simulink model "webserver_demo"  (Simulink 7.3)
settings: Solver=FixedStepDiscrete  SolverMode=SingleTasking  StartTime=0.0  StopTime=10.0  RelTol=1e-3
PreLoadFcn:
  | waijung.modelPreload; % Required for working with Waijung Blockset. Do not remove.
undefined symbols (not defined in the file): A1, A2, A7, B10, B11, B12, Blocking, C1, C2, C3, C4, C5, G14, GPIO_Pin_13, H2, H3, H6, H7, HSEOSC, Link, LQFP176, Non, ST, STM32F417IG
libraries: simulink x14, stm32f4_io_lib x4, waijung_webserver x3, amg_sqlite_dataserver x3, stm32f4_adc_lib x1, stm32f4_device_config_lib x1
(part 2 of 3)

== system webserver_demo/Http Webserver Setup ==
  Ethernet Application Setup : waijung_webserver/Ethernet Application Setup  conf=Setup  ipaddress=192.168.1.41  netmask=255.255.255.0  gateway=192.168.1.1  macaddress=02-00-00-00-00-00  dhcp=off  timerscaler=10  portpinstr=0  sampletime=0.001  blockid=HttpWebserverSetupEthernetApplicationSetup  inputporttype=[]  inputportwidth=[]  inputportlabel={}  outputporttype=[]  outputportwidth=[]  outputportlabel={}  compat=0  optionstring="[\"Dummy\",\"192\",\"168\",\"1\",\"41\",\"255\",\"255\",\"255\",\"0\",\"192\",\"168\",\"1\",\"1\",\"02\",\"00\",\"00\",\"00\",\"00\",\"00\",\"off\",\"10\"]"
  Ethernet Link Setup : waijung_webserver/Ethernet Link Setup  conf=Setup  interfacepin=Profile #2  wj_interfacetype=MII  pin_mdio=A2  pin_mdc=C1  pin_pps=Not used  pin_crs=H2  pin_col=H3  pin_dv=A7  pin_rxclk=A1  pin_rxer=B10  pin_rxd0=C4  pin_rxd1=C5  pin_rxd2=H6  pin_rxd3=H7  pin_txclk=C3  pin_txen=B11  pin_txd0=B12  pin_txd1=G14  pin_txd2=C2  pin_txd3=E2  portpinstr=H2,A1,A2,H3,A7,H6,H7,E2,B10,B11,B12,G14,C1,C2,C3,C4,C5  sampletime=inf  blockid=HttpWebserverSetupEthernetLinkSetup  inputporttype=[]  inputportwidth=[]  inputportlabel={}  outputporttype=[]  outputportwidth=[]  outputportlabel={}  compat=0  optionstring="[\"xxx\",\"on\",\"on\",\"on\",\"off\",\"on\",\"off\",\"on\",\"on\",\"off\",\"on\",\"on\",\"on\",\"on\",\"on\",\"on\",\"on\",\"off\",\"on\",\"on\",\"on\",\"on\",\"on\",\"on\",\"on\",\"on\",\"on\",\"on\",\"H\",\"2\",\"A\",\"1\",\"A\",\"2\",\"H\",\"3\",\"A\",\"7\",\"H\",\"6\",\"H\",\"7\",\"N\",\"ot used\",\"E\",\"2\",\"B\",\"10\",\"B\",\"11\",\"B\",\"12\",\"G\",\"14\",\"C\",\"1\",\"C\",\"2\",\"C\",\"3\",\"C\",\"4\",\"C\",\"5\",\"MII\"]"
  Http Server Setup : waijung_webserver/Http Server Setup  conf=Setup  port=80  ssl=Disable  sqlite=Enable  iap=Disable  mempool=8  debugport=Disable  portpinstr=0  sampletime=inf  blockid=HttpWebserverSetupHttpServerSetup  inputporttype=[]  inputportwidth=[]  inputportlabel={}  outputporttype=[]  outputportwidth=[]  outputportlabel={}  compat=0  optionstring="[\"80\",\"0\",\"0\",\"Enable\",\"Disable\",\"8\",\"17.02a\",\"\",\"\",\"\",\"adc\",\"single\",\"ADCDemoVolatileDataStorage2_adc\",\"1\",\"0\",\"0\",\"(void*)0\",\"%1.2f\",\"\",\"\",\"adc_f\",\"string\",\"ADCDemoVolatileDataStorage3_adc_f\",\"64\",\"0\",\"0\",\"(void*)0\",\"%s\",\"\",\"\",\"btn2\",\"string\",\"ButtonDemoVolatileDataStorage2_btn2\",\"4\",\"0\",\"0\",\"(void*)0\",\"%s\",\"\",\"\",\"btn3\",\"string\",\"ButtonDemoVolatileDataStorage3_btn3\",\"4\",\"0\",\"0\",\"(void*)0\",\"%s\",\"\",\"\",\"btn1\",\"string\",\"ButtonDemoVolatileDataStorage5_btn1\",\"4\",\"0\",\"0\",\"(void*)0\",\"%s\",\"\",\"\",\"dip\",\"string\",\"DIPSwitchDemoVolatileDataStorage_dip\",\"64\",\"1\",\"0\",\"(void*)0\",\"%s\",\"\",\"\",\"datetime\",\"string\",\"HighprecisionRTCDemoVolatileDataStorage1_datetime\",\"64\",\"1\",\"0\",\"(void*)0\",\"%s\",\"\",\"\",\"lcd_line2\",\"string\",\"LCDDemoVolatileDataStorage1_lcd_line2\",\"17\",\"1\",\"0\",\"(void*)0\",\"%s\",\"\",\"\",\"lcd_line3\",\"string\",\"LCDDemoVolatileDataStorage2_lcd_line3\",\"17\",\"1\",\"0\",\"(void*)0\",\"%s\",\"\",\"\",\"lcd_line4\",\"string\",\"LCDDemoVolatileDataStorage3_lcd_line4\",\"17\",\"1\",\"0\",\"(void*)0\",\"%s\",\"\",\"\",\"lcd_line1\",\"string\",\"LCDDemoVolatileDataStorage4_lcd_line1\",\"17\",\"1\",\"0\",\"(void*)0\",\"%s\",\"\",\"\",\"led1\",\"uint32\",\"LEDToggleDemoVolatileDataStorage_led1\",\"1\",\"1\",\"0\",\"LEDToggleDemoHttpserverCGIvarsetcallback_varset_ISR\",\"%u\",\"\",\"\",\"pwm\",\"uint32\",\"PWMDemoVolatileDataStorage_pwm\",\"1\",\"1\",\"0\",\"(void*)0\",\"%u\",\"\",\"\"]"

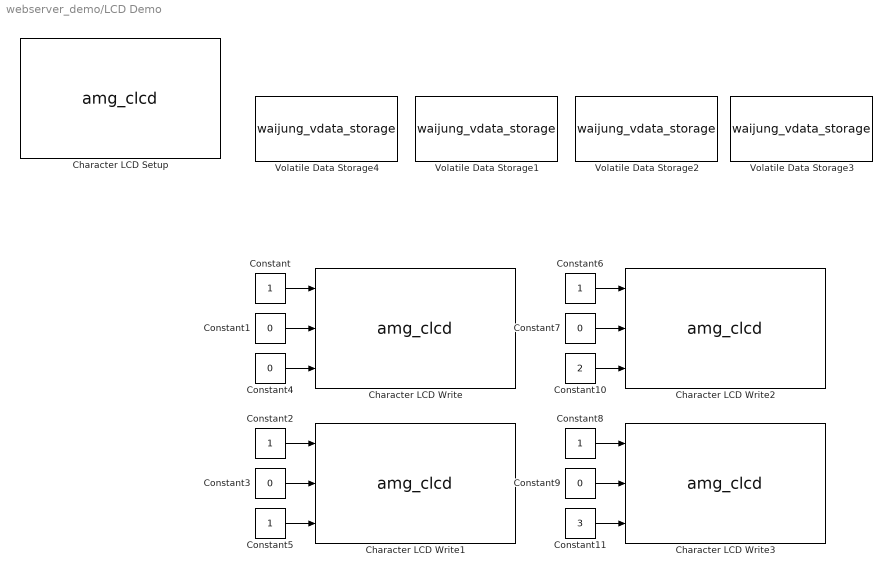
== system webserver_demo/LCD Demo ==
  Character LCD Setup : S-Function  FunctionName=amg_clcd  Parameters=module,configuration,inputtypearray,outputtypearray,confstr,sampletime,sampletimestr,blockid  EnableBusSupport=off  mask(amg_clcd){configuration=Setup, module=1, model=amg CLCD Std, interface=4-bits, linecount=4, columncount=16, gpiotype=Push-pull, controlport=E, control_rs=7, control_rw=8, control_en=9, dataport=E, data0=12, data1=13, data2=14, data3=15, usestringbuffer=off, stringbuffer=<empty>, varname=, inputtypearray=[0], outputtypearray=[0], confstr=["4","4","16","PP","E","7","9","8","","E","","","","","12","13","14","15","0","","0","0","0","0","1","0","0","0","0","stm32f4"], sampletime=-1, sampletimestr=0.001, blockid=LCDDemoCharacterLCDSetup}
      mask prompts: model "LCD model:"; linecount "Number of lines (2 or 4):"; columncount "Number of columns:"; gpiotype "GPIO Output type:"; controlport "GPIO control port:"; control_rs "GPIO control pin, RS:"; control_rw "GPIO control pin, RW:"; control_en "GPIO control pin, EN:"; dataport "GPIO data D[7:4] port"; data0 "GPIO data pin, D4:"; data1 "GPIO data pin, D5:"; data2 "GPIO data pin, D6:"; data3 "GPIO data pin, D7:"; usestringbuffer "Use string buffer"; stringbuffer "String buffer"; varname "Variable name"; inputtypearray "Input type array"; outputtypearray "Output type array"; confstr "Configuration string"; sampletime "Sample time (sec)"; sampletimestr "Compiled sample time (sec) in string"
      mask init:
      | amg_clcd_callback('init');
      mask Help: web(fullfile(waijungdocroot,'amg_clcd_setup.htm'), '-browser')
      mask StyleString: popup(Setup|Transaction),popup(1|2|3|4),popup(amg CLCD Std),popup(4-bits),edit,edit,popup(Push-pull|Open-drain),popup(A|B|C|D|E|F|G|H|I),popup(0|1|2|3|4|5|6|7|8|9|10|11|12|13|14|15),popup(0|1|2|3|4|5|6|7|8|9|10|11|12|13|14|15),popup(0|1|2|3|4|5|6|7|8|9|10|11|12|13|14|15),popup(A|B|C|D|E|F|G|H|I),popup(0|1|2|3|4|5|6|7|8|9|10|11|12|13|14|15),popup(0|1|2|3|4|5|6|7|8|9|10|11|12|13|14|15),popup(0|1|2|3|4|5|6|7|8|9|10|11|12|13|14|15),popup(0|1|2|3|4|5|6|7|8|9|10|11|12|13|14|15),checkbox,popup(<empty>),edit,edit,edit,edit,edit,edit,edit
      mask CallbackString: amg_clcd_callback('configuration');||||||||||||||||amg_clcd_callback('usestringbuffer');||amg_clcd_callback('varname');|||amg_clcd_callback('confstr');|amg_clcd_callback('sampletime');|amg_clcd_callback('sampletimestr');|amg_clcd_callback('blockid');
      mask Display: text(0.5, 0.5, 'Module: CLCD1 (Setup)\nInterface: 4-bits\nCntrl: E7/E8/E9\nD[7:4]: E12/E13/E14/E15\nTs (sec): 0.001','ver','middle','hor','center');
  Character LCD Write : S-Function  FunctionName=amg_clcd  Parameters=module,configuration,inputtypearray,outputtypearray,confstr,sampletime,sampletimestr,blockid  EnableBusSupport=off  mask(amg_clcd){configuration=Transaction, module=1, model=amg CLCD Std, interface=4-bits, linecount=4, columncount=20, gpiotype=Push-pull, controlport=E, control_rs=15, control_rw=13, control_en=11, dataport=A, data0=7, data1=5, data2=3, data3=1, usestringbuffer=on, stringbuffer=lcd_line1, varname=LCDDemoVolatileDataStorage4_lcd_line1, inputtypearray=[3 -1 -1 -1], outputtypearray=[0], confstr=["4","4","20","PP","E","15","11","13","","A","","","","","7","5","3","1","1","LCDDemoVolatileDataStorage4_lcd_line1","1","0","0","0","1","0","0","0","0","stm32f4"], sampletime=-1, sampletimestr=0.001, blockid=LCDDemoCharacterLCDWrite}
      mask prompts: model "LCD model:"; linecount "Number of lines:"; columncount "Number of columns:"; gpiotype "GPIO Output type:"; controlport "GPIO control port:"; control_rs "GPIO control pin, RS:"; control_rw "GPIO control pin, RW:"; control_en "GPIO control pin, EN:"; dataport "GPIO data D[7:4] port"; data0 "GPIO data pin, D4:"; data1 "GPIO data pin, D5:"; data2 "GPIO data pin, D6:"; data3 "GPIO data pin, D7:"; usestringbuffer "Use string buffer"; stringbuffer "String buffer"; varname "Variable name"; inputtypearray "Input type array"; outputtypearray "Output type array"; confstr "Configuration string"; sampletime "Sample time (sec)"; sampletimestr "Compiled sample time (sec) in string"
      mask help:
      | Note for cmd:
      | 1 - Clear LCD Line before write.
      | 0 or otherwise - Write into LCD Line with existing data.
      mask init:
      | amg_clcd_callback('init');
      mask Help: web(fullfile(waijungdocroot,'amg_clcd_write.htm'), '-browser')
      mask StyleString: popup(Setup|Transaction),popup(1|2|3|4),popup(amg CLCD Std),popup(4-bits),edit,edit,popup(Push-pull|Open-drain),popup(A|B|C|D|E|F|G|H|I),popup(0|1|2|3|4|5|6|7|8|9|10|11|12|13|14|15),popup(0|1|2|3|4|5|6|7|8|9|10|11|12|13|14|15),popup(0|1|2|3|4|5|6|7|8|9|10|11|12|13|14|15),popup(A|B|C|D|E|F|G|H|I),popup(0|1|2|3|4|5|6|7|8|9|10|11|12|13|14|15),popup(0|1|2|3|4|5|6|7|8|9|10|11|12|13|14|15),popup(0|1|2|3|4|5|6|7|8|9|10|11|12|13|14|15),popup(0|1|2|3|4|5|6|7|8|9|10|11|12|13|14|15),checkbox,popup(adc_f|button_on|button_off|btn2|btn3|btn1|dip|datetime|lcd_line2|lcd_line3|lcd_line4|lcd_line1),edit,edit,edit,edit,edit,edit,edit
      mask CallbackString: amg_clcd_callback('configuration');||||||||||||||||amg_clcd_callback('usestringbuffer');||amg_clcd_callback('varname');|||amg_clcd_callback('confstr');|amg_clcd_callback('sampletime');|amg_clcd_callback('sampletimestr');|amg_clcd_callback('blockid');
      mask Display: text(0.5, 0.5, 'Module: CLCD1 (Write)\nBuffer: lcd_line1\nTs (sec): 0.001','ver','middle','hor','center');port_label('input', 1,'cmd');port_label('input', 2,'xpos');port_label('input', 3,'ypos');
  Character LCD Write1 : S-Function  FunctionName=amg_clcd  Parameters=module,configuration,inputtypearray,outputtypearray,confstr,sampletime,sampletimestr,blockid  EnableBusSupport=off  mask(amg_clcd){configuration=Transaction, module=1, model=amg CLCD Std, interface=4-bits, linecount=4, columncount=20, gpiotype=Push-pull, controlport=E, control_rs=15, control_rw=13, control_en=11, dataport=A, data0=7, data1=5, data2=3, data3=1, usestringbuffer=on, stringbuffer=lcd_line2, varname=LCDDemoVolatileDataStorage1_lcd_line2, inputtypearray=[3 -1 -1 -1], outputtypearray=[0], confstr=["4","4","20","PP","E","15","11","13","","A","","","","","7","5","3","1","1","LCDDemoVolatileDataStorage1_lcd_line2","1","0","0","0","1","0","0","0","0","stm32f4"], sampletime=-1, sampletimestr=0.001, blockid=LCDDemoCharacterLCDWrite1}
      mask prompts: model "LCD model:"; linecount "Number of lines:"; columncount "Number of columns:"; gpiotype "GPIO Output type:"; controlport "GPIO control port:"; control_rs "GPIO control pin, RS:"; control_rw "GPIO control pin, RW:"; control_en "GPIO control pin, EN:"; dataport "GPIO data D[7:4] port"; data0 "GPIO data pin, D4:"; data1 "GPIO data pin, D5:"; data2 "GPIO data pin, D6:"; data3 "GPIO data pin, D7:"; usestringbuffer "Use string buffer"; stringbuffer "String buffer"; varname "Variable name"; inputtypearray "Input type array"; outputtypearray "Output type array"; confstr "Configuration string"; sampletime "Sample time (sec)"; sampletimestr "Compiled sample time (sec) in string"
      mask help:
      | Note for cmd:
      | 1 - Clear LCD Line before write.
      | 0 or otherwise - Write into LCD Line with existing data.
      mask init:
      | amg_clcd_callback('init');
      mask Help: web(fullfile(waijungdocroot,'amg_clcd_write.htm'), '-browser')
      mask StyleString: popup(Setup|Transaction),popup(1|2|3|4),popup(amg CLCD Std),popup(4-bits),edit,edit,popup(Push-pull|Open-drain),popup(A|B|C|D|E|F|G|H|I),popup(0|1|2|3|4|5|6|7|8|9|10|11|12|13|14|15),popup(0|1|2|3|4|5|6|7|8|9|10|11|12|13|14|15),popup(0|1|2|3|4|5|6|7|8|9|10|11|12|13|14|15),popup(A|B|C|D|E|F|G|H|I),popup(0|1|2|3|4|5|6|7|8|9|10|11|12|13|14|15),popup(0|1|2|3|4|5|6|7|8|9|10|11|12|13|14|15),popup(0|1|2|3|4|5|6|7|8|9|10|11|12|13|14|15),popup(0|1|2|3|4|5|6|7|8|9|10|11|12|13|14|15),checkbox,popup(adc_f|button_on|button_off|btn2|btn3|btn1|dip|datetime|lcd_line2|lcd_line3|lcd_line4|lcd_line1),edit,edit,edit,edit,edit,edit,edit
      mask CallbackString: amg_clcd_callback('configuration');||||||||||||||||amg_clcd_callback('usestringbuffer');||amg_clcd_callback('varname');|||amg_clcd_callback('confstr');|amg_clcd_callback('sampletime');|amg_clcd_callback('sampletimestr');|amg_clcd_callback('blockid');
      mask Display: text(0.5, 0.5, 'Module: CLCD1 (Write)\nBuffer: lcd_line2\nTs (sec): 0.001','ver','middle','hor','center');port_label('input', 1,'cmd');port_label('input', 2,'xpos');port_label('input', 3,'ypos');
  Character LCD Write2 : S-Function  FunctionName=amg_clcd  Parameters=module,configuration,inputtypearray,outputtypearray,confstr,sampletime,sampletimestr,blockid  EnableBusSupport=off  mask(amg_clcd){configuration=Transaction, module=1, model=amg CLCD Std, interface=4-bits, linecount=4, columncount=20, gpiotype=Push-pull, controlport=E, control_rs=15, control_rw=13, control_en=11, dataport=A, data0=7, data1=5, data2=3, data3=1, usestringbuffer=on, stringbuffer=lcd_line3, varname=LCDDemoVolatileDataStorage2_lcd_line3, inputtypearray=[3 -1 -1 -1], outputtypearray=[0], confstr=["4","4","20","PP","E","15","11","13","","A","","","","","7","5","3","1","1","LCDDemoVolatileDataStorage2_lcd_line3","1","0","0","0","1","0","0","0","0","stm32f4"], sampletime=-1, sampletimestr=0.001, blockid=LCDDemoCharacterLCDWrite2}
      mask prompts: model "LCD model:"; linecount "Number of lines:"; columncount "Number of columns:"; gpiotype "GPIO Output type:"; controlport "GPIO control port:"; control_rs "GPIO control pin, RS:"; control_rw "GPIO control pin, RW:"; control_en "GPIO control pin, EN:"; dataport "GPIO data D[7:4] port"; data0 "GPIO data pin, D4:"; data1 "GPIO data pin, D5:"; data2 "GPIO data pin, D6:"; data3 "GPIO data pin, D7:"; usestringbuffer "Use string buffer"; stringbuffer "String buffer"; varname "Variable name"; inputtypearray "Input type array"; outputtypearray "Output type array"; confstr "Configuration string"; sampletime "Sample time (sec)"; sampletimestr "Compiled sample time (sec) in string"
      mask help:
      | Note for cmd:
      | 1 - Clear LCD Line before write.
      | 0 or otherwise - Write into LCD Line with existing data.
      mask init:
      | amg_clcd_callback('init');
      mask Help: web(fullfile(waijungdocroot,'amg_clcd_write.htm'), '-browser')
      mask StyleString: popup(Setup|Transaction),popup(1|2|3|4),popup(amg CLCD Std),popup(4-bits),edit,edit,popup(Push-pull|Open-drain),popup(A|B|C|D|E|F|G|H|I),popup(0|1|2|3|4|5|6|7|8|9|10|11|12|13|14|15),popup(0|1|2|3|4|5|6|7|8|9|10|11|12|13|14|15),popup(0|1|2|3|4|5|6|7|8|9|10|11|12|13|14|15),popup(A|B|C|D|E|F|G|H|I),popup(0|1|2|3|4|5|6|7|8|9|10|11|12|13|14|15),popup(0|1|2|3|4|5|6|7|8|9|10|11|12|13|14|15),popup(0|1|2|3|4|5|6|7|8|9|10|11|12|13|14|15),popup(0|1|2|3|4|5|6|7|8|9|10|11|12|13|14|15),checkbox,popup(adc_f|button_on|button_off|btn2|btn3|btn1|dip|datetime|lcd_line2|lcd_line3|lcd_line4|lcd_line1),edit,edit,edit,edit,edit,edit,edit
      mask CallbackString: amg_clcd_callback('configuration');||||||||||||||||amg_clcd_callback('usestringbuffer');||amg_clcd_callback('varname');|||amg_clcd_callback('confstr');|amg_clcd_callback('sampletime');|amg_clcd_callback('sampletimestr');|amg_clcd_callback('blockid');
      mask Display: text(0.5, 0.5, 'Module: CLCD1 (Write)\nBuffer: lcd_line3\nTs (sec): 0.001','ver','middle','hor','center');port_label('input', 1,'cmd');port_label('input', 2,'xpos');port_label('input', 3,'ypos');
  Character LCD Write3 : S-Function  FunctionName=amg_clcd  Parameters=module,configuration,inputtypearray,outputtypearray,confstr,sampletime,sampletimestr,blockid  EnableBusSupport=off  mask(amg_clcd){configuration=Transaction, module=1, model=amg CLCD Std, interface=4-bits, linecount=4, columncount=20, gpiotype=Push-pull, controlport=E, control_rs=15, control_rw=13, control_en=11, dataport=A, data0=7, data1=5, data2=3, data3=1, usestringbuffer=on, stringbuffer=lcd_line4, varname=LCDDemoVolatileDataStorage3_lcd_line4, inputtypearray=[3 -1 -1 -1], outputtypearray=[0], confstr=["4","4","20","PP","E","15","11","13","","A","","","","","7","5","3","1","1","LCDDemoVolatileDataStorage3_lcd_line4","1","0","0","0","1","0","0","0","0","stm32f4"], sampletime=-1, sampletimestr=0.001, blockid=LCDDemoCharacterLCDWrite3}
      mask prompts: model "LCD model:"; linecount "Number of lines:"; columncount "Number of columns:"; gpiotype "GPIO Output type:"; controlport "GPIO control port:"; control_rs "GPIO control pin, RS:"; control_rw "GPIO control pin, RW:"; control_en "GPIO control pin, EN:"; dataport "GPIO data D[7:4] port"; data0 "GPIO data pin, D4:"; data1 "GPIO data pin, D5:"; data2 "GPIO data pin, D6:"; data3 "GPIO data pin, D7:"; usestringbuffer "Use string buffer"; stringbuffer "String buffer"; varname "Variable name"; inputtypearray "Input type array"; outputtypearray "Output type array"; confstr "Configuration string"; sampletime "Sample time (sec)"; sampletimestr "Compiled sample time (sec) in string"
      mask help:
      | Note for cmd:
      | 1 - Clear LCD Line before write.
      | 0 or otherwise - Write into LCD Line with existing data.
      mask init:
      | amg_clcd_callback('init');
      mask Help: web(fullfile(waijungdocroot,'amg_clcd_write.htm'), '-browser')
      mask StyleString: popup(Setup|Transaction),popup(1|2|3|4),popup(amg CLCD Std),popup(4-bits),edit,edit,popup(Push-pull|Open-drain),popup(A|B|C|D|E|F|G|H|I),popup(0|1|2|3|4|5|6|7|8|9|10|11|12|13|14|15),popup(0|1|2|3|4|5|6|7|8|9|10|11|12|13|14|15),popup(0|1|2|3|4|5|6|7|8|9|10|11|12|13|14|15),popup(A|B|C|D|E|F|G|H|I),popup(0|1|2|3|4|5|6|7|8|9|10|11|12|13|14|15),popup(0|1|2|3|4|5|6|7|8|9|10|11|12|13|14|15),popup(0|1|2|3|4|5|6|7|8|9|10|11|12|13|14|15),popup(0|1|2|3|4|5|6|7|8|9|10|11|12|13|14|15),checkbox,popup(adc_f|button_on|button_off|btn2|btn3|btn1|dip|datetime|lcd_line2|lcd_line3|lcd_line4|lcd_line1),edit,edit,edit,edit,edit,edit,edit
      mask CallbackString: amg_clcd_callback('configuration');||||||||||||||||amg_clcd_callback('usestringbuffer');||amg_clcd_callback('varname');|||amg_clcd_callback('confstr');|amg_clcd_callback('sampletime');|amg_clcd_callback('sampletimestr');|amg_clcd_callback('blockid');
      mask Display: text(0.5, 0.5, 'Module: CLCD1 (Write)\nBuffer: lcd_line4\nTs (sec): 0.001','ver','middle','hor','center');port_label('input', 1,'cmd');port_label('input', 2,'xpos');port_label('input', 3,'ypos');
  Constant{,2,5..6,8} (5 alike) : Constant  OutDataTypeMode=uint8  OutDataType=fixdt(1, 16)  OutScaling=2^0  OutDataTypeStr=uint8
  Constant{1,3..4,7,9} (5 alike) : Constant  Value=0  OutDataTypeMode=uint8  OutDataType=fixdt(1, 16)  OutScaling=2^0  OutDataTypeStr=uint8
  Constant10 : Constant  Value=2  OutDataTypeMode=uint8  OutDataType=fixdt(1, 16)  OutScaling=2^0  OutDataTypeStr=uint8
  Constant11 : Constant  Value=3  OutDataTypeMode=uint8  OutDataType=fixdt(1, 16)  OutScaling=2^0  OutDataTypeStr=uint8
  Volatile Data Storage1 : S-Function  FunctionName=waijung_vdata_storage  Parameters=storagetype,storagename,initval,varname,buffersize,initvalstring,sampletime,sampletimestr,blockid,storagetypestr  EnableBusSupport=off  mask(waijung_vdata_storage){storagetype=string, storagename=lcd_line2, initval=0, varname=LCDDemoVolatileDataStorage1_lcd_line2, buffersize=17, initvalstring='', webintegration=Write/ Read, weboutputformat='%s', webcgicallback=(void*)0, sampletime=-1, sampletimestr=0.001, blockid=LCDDemoVolatileDataStorage1, storagetypestr=char}
      mask prompts: storagetype "Storage Type"; storagename "Storage Name (must be a valid variable name)"; initval "Initial value (Apply at Power on Reset only)"; varname "Variable name"; buffersize "Size (bytes)"; initvalstring "Initial value (Apply at Power on Reset only)"; webintegration "Web CGI varget/varset integration"; weboutputformat "Web CGI varget output format"; webcgicallback "Web CGI varset callback"; sampletime "Sample time (sec)"; sampletimestr "Compiled sample time (sec) in string"; storagetypestr "Type string"
      mask help: This block implements a volatile Data Storage.
      mask init:
      | waijung_vdata_storage_callback('init');
      mask Help: web(fullfile(waijungdocroot,'Volatile_Data_Storage.htm'))
      mask StyleString: popup(double|single|uint32|int32|uint16|int16|uint8|int8|string),edit,edit,edit,edit,edit,popup(Disable|ReadOnly|Write/ Read|ReadOnly with KeyValuePair|Write/ Read with KeyValuePair),edit,edit,edit,edit,edit,edit
      mask CallbackString: waijung_vdata_storage_callback('storagetype');|waijung_vdata_storage_callback('storagename');|waijung_vdata_storage_callback('initval');|waijung_vdata_storage_callback('varname');||waijung_vdata_storage_callback('initvalstring');|waijung_vdata_storage_callback('webintegration');|waijung_vdata_storage_callback('weboutputformat');||waijung_vdata_storage_callback('sampletime');|waijung_vdata_storage_callback('sampletimestr');|waijung_vdata_storage_callback('blockid');|
      mask Display: text(0.5, 0.5, 'Name: lcd_line2\nType: string','ver','middle','hor','center')
  Volatile Data Storage2 : S-Function  FunctionName=waijung_vdata_storage  Parameters=storagetype,storagename,initval,varname,buffersize,initvalstring,sampletime,sampletimestr,blockid,storagetypestr  EnableBusSupport=off  mask(waijung_vdata_storage){storagetype=string, storagename=lcd_line3, initval=0, varname=LCDDemoVolatileDataStorage2_lcd_line3, buffersize=17, initvalstring='', webintegration=Write/ Read, weboutputformat='%s', webcgicallback=(void*)0, sampletime=-1, sampletimestr=0.001, blockid=LCDDemoVolatileDataStorage2, storagetypestr=char}
      mask prompts: storagetype "Storage Type"; storagename "Storage Name (must be a valid variable name)"; initval "Initial value (Apply at Power on Reset only)"; varname "Variable name"; buffersize "Size (bytes)"; initvalstring "Initial value (Apply at Power on Reset only)"; webintegration "Web CGI varget/varset integration"; weboutputformat "Web CGI varget output format"; webcgicallback "Web CGI varset callback"; sampletime "Sample time (sec)"; sampletimestr "Compiled sample time (sec) in string"; storagetypestr "Type string"
      mask help: This block implements a volatile Data Storage.
      mask init:
      | waijung_vdata_storage_callback('init');
      mask Help: web(fullfile(waijungdocroot,'Volatile_Data_Storage.htm'))
      mask StyleString: popup(double|single|uint32|int32|uint16|int16|uint8|int8|string),edit,edit,edit,edit,edit,popup(Disable|ReadOnly|Write/ Read|ReadOnly with KeyValuePair|Write/ Read with KeyValuePair),edit,edit,edit,edit,edit,edit
      mask CallbackString: waijung_vdata_storage_callback('storagetype');|waijung_vdata_storage_callback('storagename');|waijung_vdata_storage_callback('initval');|waijung_vdata_storage_callback('varname');||waijung_vdata_storage_callback('initvalstring');|waijung_vdata_storage_callback('webintegration');|waijung_vdata_storage_callback('weboutputformat');||waijung_vdata_storage_callback('sampletime');|waijung_vdata_storage_callback('sampletimestr');|waijung_vdata_storage_callback('blockid');|
      mask Display: text(0.5, 0.5, 'Name: lcd_line3\nType: string','ver','middle','hor','center')
  Volatile Data Storage3 : S-Function  FunctionName=waijung_vdata_storage  Parameters=storagetype,storagename,initval,varname,buffersize,initvalstring,sampletime,sampletimestr,blockid,storagetypestr  EnableBusSupport=off  mask(waijung_vdata_storage){storagetype=string, storagename=lcd_line4, initval=0, varname=LCDDemoVolatileDataStorage3_lcd_line4, buffersize=17, initvalstring='', webintegration=Write/ Read, weboutputformat='%s', webcgicallback=(void*)0, sampletime=-1, sampletimestr=0.001, blockid=LCDDemoVolatileDataStorage3, storagetypestr=char}
      mask prompts: storagetype "Storage Type"; storagename "Storage Name (must be a valid variable name)"; initval "Initial value (Apply at Power on Reset only)"; varname "Variable name"; buffersize "Size (bytes)"; initvalstring "Initial value (Apply at Power on Reset only)"; webintegration "Web CGI varget/varset integration"; weboutputformat "Web CGI varget output format"; webcgicallback "Web CGI varset callback"; sampletime "Sample time (sec)"; sampletimestr "Compiled sample time (sec) in string"; storagetypestr "Type string"
      mask help: This block implements a volatile Data Storage.
      mask init:
      | waijung_vdata_storage_callback('init');
      mask Help: web(fullfile(waijungdocroot,'Volatile_Data_Storage.htm'))
      mask StyleString: popup(double|single|uint32|int32|uint16|int16|uint8|int8|string),edit,edit,edit,edit,edit,popup(Disable|ReadOnly|Write/ Read|ReadOnly with KeyValuePair|Write/ Read with KeyValuePair),edit,edit,edit,edit,edit,edit
      mask CallbackString: waijung_vdata_storage_callback('storagetype');|waijung_vdata_storage_callback('storagename');|waijung_vdata_storage_callback('initval');|waijung_vdata_storage_callback('varname');||waijung_vdata_storage_callback('initvalstring');|waijung_vdata_storage_callback('webintegration');|waijung_vdata_storage_callback('weboutputformat');||waijung_vdata_storage_callback('sampletime');|waijung_vdata_storage_callback('sampletimestr');|waijung_vdata_storage_callback('blockid');|
      mask Display: text(0.5, 0.5, 'Name: lcd_line4\nType: string','ver','middle','hor','center')
  Volatile Data Storage4 : S-Function  FunctionName=waijung_vdata_storage  Parameters=storagetype,storagename,initval,varname,buffersize,initvalstring,sampletime,sampletimestr,blockid,storagetypestr  EnableBusSupport=off  mask(waijung_vdata_storage){storagetype=string, storagename=lcd_line1, initval=0, varname=LCDDemoVolatileDataStorage4_lcd_line1, buffersize=17, initvalstring='Welcome', webintegration=Write/ Read, weboutputformat='%s', webcgicallback=(void*)0, sampletime=-1, sampletimestr=0.001, blockid=LCDDemoVolatileDataStorage4, storagetypestr=char}
      mask prompts: storagetype "Storage Type"; storagename "Storage Name (must be a valid variable name)"; initval "Initial value (Apply at Power on Reset only)"; varname "Variable name"; buffersize "Size (bytes)"; initvalstring "Initial value (Apply at Power on Reset only)"; webintegration "Web CGI varget/varset integration"; weboutputformat "Web CGI varget output format"; webcgicallback "Web CGI varset callback"; sampletime "Sample time (sec)"; sampletimestr "Compiled sample time (sec) in string"; storagetypestr "Type string"
      mask help: This block implements a volatile Data Storage.
      mask init:
      | waijung_vdata_storage_callback('init');
      mask Help: web(fullfile(waijungdocroot,'Volatile_Data_Storage.htm'))
      mask StyleString: popup(double|single|uint32|int32|uint16|int16|uint8|int8|string),edit,edit,edit,edit,edit,popup(Disable|ReadOnly|Write/ Read|ReadOnly with KeyValuePair|Write/ Read with KeyValuePair),edit,edit,edit,edit,edit,edit
      mask CallbackString: waijung_vdata_storage_callback('storagetype');|waijung_vdata_storage_callback('storagename');|waijung_vdata_storage_callback('initval');|waijung_vdata_storage_callback('varname');||waijung_vdata_storage_callback('initvalstring');|waijung_vdata_storage_callback('webintegration');|waijung_vdata_storage_callback('weboutputformat');||waijung_vdata_storage_callback('sampletime');|waijung_vdata_storage_callback('sampletimestr');|waijung_vdata_storage_callback('blockid');|
      mask Display: text(0.5, 0.5, 'Name: lcd_line1\nType: string','ver','middle','hor','center')
  wires:
  Constant/1 -> Character LCD Write/1
  Constant1/1 -> Character LCD Write/2
  Constant2/1 -> Character LCD Write1/1
  Constant3/1 -> Character LCD Write1/2
  Constant4/1 -> Character LCD Write/3
  Constant5/1 -> Character LCD Write1/3
  Constant6/1 -> Character LCD Write2/1
  Constant7/1 -> Character LCD Write2/2
  Constant8/1 -> Character LCD Write3/1
  Constant9/1 -> Character LCD Write3/2
  Constant10/1 -> Character LCD Write2/3
  Constant11/1 -> Character LCD Write3/3

== system webserver_demo/LED Toggle Demo ==
  Function-Call Subsystem : Subsystem  TreatAsAtomicUnit=on
  Httpserver CGI varset callback : S-Function  FunctionName=waijung_webserver_vdata_mapping  Parameters=callback,inputtype,outputtype,sampletime,blockid  EnableBusSupport=off  mask(waijung_webserver_vdata_mapping){vdatamapping=led1, vdatareference=LEDToggleDemoVolatileDataStorage_led1, vdatatype=uint32, vdatasize=1, accessmode=ReadWrite, callback=on, namevaluepair=on, callbackisr=LEDToggleDemoHttpserverCGIvarsetcallback_varset_ISR, obsoletestatus=No, inputtype=[0], outputtype=[0], blockid=LEDToggleDemoHttpserverCGIvarsetcallback, sampletime=inf}
      mask prompts: vdatamapping "Volatile Data Mapping"; vdatareference "Volatile Data Reference"; vdatatype "Data type"; vdatasize "Size"; accessmode "Access mode"; callback "Enable callback on CGI varset"; namevaluepair "Enable 'name=value' pair on CGI varget"; callbackisr "Callback ISR"; obsoletestatus "Obsolete status"; inputtype "Input data type"; outputtype "Output data type"; sampletime "Sample time (sec)"
      mask help: The block generate function-call during variable set value via http varset.cgi
      mask init:
      | waijung_webserver_vdata_mapping_callback('init');
      mask Help: web(fullfile(waijungdocroot,'Webserver_Volatile_Data_Mappin.htm'), '-browser')
      mask StyleString: popup(adc|adc_f|button_on|button_off|btn2|btn3|btn1|dip|datetime|lcd_line2|lcd_line3|lcd_line4|lcd_line1|led1|pwm),edit,edit,edit,popup(ReadWrite|ReadOnly),checkbox,checkbox,edit,popup(No),edit,edit,edit,edit
      mask CallbackString: waijung_webserver_vdata_mapping_callback('vdatamapping');||||waijung_webserver_vdata_mapping_callback('accessmode');|||||||waijung_webserver_vdata_mapping_callback('blockid');|
      mask Display: text(0.05, 0.5, 'Mapping: led1\nAccess: ReadWrite','ver','middle','hor','left');port_label('output', 1,'Call ISR');
  Volatile Data Storage : S-Function  FunctionName=waijung_vdata_storage  Parameters=storagetype,storagename,initval,varname,buffersize,initvalstring,sampletime,sampletimestr,blockid,storagetypestr  EnableBusSupport=off  mask(waijung_vdata_storage){storagetype=uint32, storagename=led1, initval=0, varname=LEDToggleDemoVolatileDataStorage_led1, buffersize=64, initvalstring='Initial string', webintegration=Write/ Read, weboutputformat='%u', webcgicallback=LEDToggleDemoHttpserverCGIvarsetcallback_varset_ISR, sampletime=-1, sampletimestr=0.001, blockid=LEDToggleDemoVolatileDataStorage, storagetypestr=uint32_t}
      mask prompts: storagetype "Storage Type"; storagename "Storage Name (must be a valid variable name)"; initval "Initial value (Apply at Power on Reset only)"; varname "Variable name"; buffersize "Size (bytes)"; initvalstring "Initial value (Apply at Power on Reset only)"; webintegration "Web CGI varget/varset integration"; weboutputformat "Web CGI varget output format"; webcgicallback "Web CGI varset callback"; sampletime "Sample time (sec)"; sampletimestr "Compiled sample time (sec) in string"; storagetypestr "Type string"
      mask help: This block implements a volatile Data Storage.
      mask init:
      | waijung_vdata_storage_callback('init');
      mask Help: web(fullfile(waijungdocroot,'Volatile_Data_Storage.htm'))
      mask StyleString: popup(double|single|uint32|int32|uint16|int16|uint8|int8|string),edit,edit,edit,edit,edit,popup(Disable|ReadOnly|Write/ Read|ReadOnly with KeyValuePair|Write/ Read with KeyValuePair),edit,edit,edit,edit,edit,edit
      mask CallbackString: waijung_vdata_storage_callback('storagetype');|waijung_vdata_storage_callback('storagename');|waijung_vdata_storage_callback('initval');|waijung_vdata_storage_callback('varname');||waijung_vdata_storage_callback('initvalstring');|waijung_vdata_storage_callback('webintegration');|waijung_vdata_storage_callback('weboutputformat');||waijung_vdata_storage_callback('sampletime');|waijung_vdata_storage_callback('sampletimestr');|waijung_vdata_storage_callback('blockid');|
      mask Display: text(0.5, 0.5, 'Name: led1\nType: uint32','ver','middle','hor','center')
  wires:
  Httpserver CGI varset callback/1 -> Function-Call Subsystem/Trigger

== system webserver_demo/PWM Demo ==
  Basic PWM : S-Function  FunctionName=stm32f4_basicpwm  Parameters=timer,pwmperiod,ch1pin,ch2pin,ch3pin,ch4pin,sampletime,sampletimestr,blockid,apb,portstr,pinstr,pinmat,timarr,timprescale,chmat,polaritystr  EnableBusSupport=off  mask(stm32f4_basicpwm){timer=4, pwmperiod=0.02, polarity=Active High, polaritystr=TIM_OCPolarity_High, ch1pin=D12, ch2pin=D13, ch3pin=Not available - Do not use, ch4pin=Not available - Do not use, sampletime=0.01, sampletimestr=0.01, blockid=PWMDemoBasicPWM, portpinstr=D12,D13,,, enablecustomportlabel=off, cinputportlabel=In1, In2, In3, In4, coutputportlabel=0, apb=1, portstr=["D"], pinstr=["GPIO_Pin_12 | GPIO_Pin_13"], pinmat=[2 12 13], timarr=64614, timprescale=25, chmat=[1  2]}
      mask prompts: pwmperiod "PWM Period (seconds)"; ch1pin "Channel 1"; ch2pin "Channel 2"; ch3pin "Channel 3"; ch4pin "Channel 4"; sampletime "Sample time (sec)"; sampletimestr "Compiled sample time (sec) in string"; portpinstr "Port pin string"; enablecustomportlabel "Enable custom port labels"; cinputportlabel "Custom input port labels (Ex. In1, In2, In3)"; coutputportlabel "Custom output port labels (Ex. Out1, Out2, Out3)"; portstr "Port string"; pinstr "Pin string"; pinmat "Pin matrix"; timarr "Timer ARR"; timprescale "Timer PRESCALE"; chmat "Channel order"
      mask help:
      | This block implements basic Edge-aligned Pulse Width Modulation (PWM) generation.
      | All timers are 16-bit. The PWM period is fixed (per timer).
      mask init:
      | stm32f4_basicpwm_callback('init');
      mask Help: web(fullfile(waijungdocroot,'stm32f4_basicpwm.htm'),'-browser')
      mask StyleString: popup(1|2|3|4|5|8|9|10|11|12|13|14),edit,popup(Active High|Active Low),edit,popup(Not available - Do not use|D12|B6),popup(Not available - Do not use|D13|B7),popup(Not available - Do not use|D14|B8),popup(Not available - Do not use|D15|B9),edit,edit,edit,edit,checkbox,edit,edit,edit,edit,edit,edit,edit,edit,edit
      mask CallbackString: stm32f4_basicpwm_callback('timer');|stm32f4_basicpwm_callback('pwmperiod');|stm32f4_basicpwm_callback('polarity');||stm32f4_basicpwm_callback('ch1pin');|stm32f4_basicpwm_callback('ch2pin');|stm32f4_basicpwm_callback('ch3pin');|stm32f4_basicpwm_callback('ch4pin');|stm32f4_basicpwm_callback('sampletime');|stm32f4_basicpwm_callback('sampletimestr');|stm32f4_basicpwm_callback('blockid');||stm32f4_basicpwm_callback('enablecustomportlabel');|||||||||
      mask Display: text(0.95, 0.5, 'Timer: 4\nPolarity: Active High\nPeriod (sec) 0.02\nTs (sec): 0.01','ver','middle','hor','right');port_label('input', 1,'CH1 (D12)');port_label('input', 2,'CH2 (D13)')
  Data Type Conversion : DataTypeConversion  OutDataType=fixdt(1, 16)  OutScaling=2^0
  Volatile Data Storage : S-Function  FunctionName=waijung_vdata_storage  Parameters=storagetype,storagename,initval,varname,buffersize,initvalstring,sampletime,sampletimestr,blockid,storagetypestr  EnableBusSupport=off  mask(waijung_vdata_storage){storagetype=uint32, storagename=pwm, initval=0, varname=PWMDemoVolatileDataStorage_pwm, buffersize=64, initvalstring='Initial string', webintegration=Write/ Read, weboutputformat='%u', webcgicallback=(void*)0, sampletime=-1, sampletimestr=0.001, blockid=PWMDemoVolatileDataStorage, storagetypestr=uint32_t}
      mask prompts: storagetype "Storage Type"; storagename "Storage Name (must be a valid variable name)"; initval "Initial value (Apply at Power on Reset only)"; varname "Variable name"; buffersize "Size (bytes)"; initvalstring "Initial value (Apply at Power on Reset only)"; webintegration "Web CGI varget/varset integration"; weboutputformat "Web CGI varget output format"; webcgicallback "Web CGI varset callback"; sampletime "Sample time (sec)"; sampletimestr "Compiled sample time (sec) in string"; storagetypestr "Type string"
      mask help: This block implements a volatile Data Storage.
      mask init:
      | waijung_vdata_storage_callback('init');
      mask Help: web(fullfile(waijungdocroot,'Volatile_Data_Storage.htm'))
      mask StyleString: popup(double|single|uint32|int32|uint16|int16|uint8|int8|string),edit,edit,edit,edit,edit,popup(Disable|ReadOnly|Write/ Read|ReadOnly with KeyValuePair|Write/ Read with KeyValuePair),edit,edit,edit,edit,edit,edit
      mask CallbackString: waijung_vdata_storage_callback('storagetype');|waijung_vdata_storage_callback('storagename');|waijung_vdata_storage_callback('initval');|waijung_vdata_storage_callback('varname');||waijung_vdata_storage_callback('initvalstring');|waijung_vdata_storage_callback('webintegration');|waijung_vdata_storage_callback('weboutputformat');||waijung_vdata_storage_callback('sampletime');|waijung_vdata_storage_callback('sampletimestr');|waijung_vdata_storage_callback('blockid');|
      mask Display: text(0.5, 0.5, 'Name: pwm\nType: uint32','ver','middle','hor','center')
  Volatile Data Storage Read : S-Function  FunctionName=waijung_vdata_read  Parameters=storagename,varname,sampletime,sampletimestr,blockid,storagetype,storagetypestr  EnableBusSupport=off  mask(waijung_vdata_read){storagename=pwm, varname=PWMDemoVolatileDataStorage_pwm, sampletime=inf, sampletimestr=0.01, blockid=PWMDemoVolatileDataStorageRead, storagetype=uint32, storagetypestr=uint32_t}
      mask prompts: storagename "Storage Name"; varname "Variable name"; sampletime "Sample time (sec)"; sampletimestr "Compiled sample time (sec) in string"; storagetype "Data type"; storagetypestr "Data type string"
      mask help: This block implements read data from a buffer.
      mask init:
      | waijung_vdata_read_callback('init');
      mask Help: web(fullfile(waijungdocroot,'waijung_vdata_read.htm'))
      mask StyleString: popup(adc|adc_f|button_on|button_off|btn2|btn3|btn1|dip|datetime|lcd_line2|lcd_line3|lcd_line4|lcd_line1|led1|pwm),edit,edit,edit,edit,edit,edit
      mask CallbackString: waijung_vdata_read_callback('storagename');|waijung_vdata_read_callback('varname');|waijung_vdata_read_callback('sampletime');|waijung_vdata_read_callback('sampletimestr');|waijung_vdata_read_callback('blockid');|waijung_vdata_read_callback('storagetype');|
      mask Display: text(0.05, 0.5, 'Buffer: pwm','ver','middle','hor','left');port_label('output',1,'D1(uint32)')
  wires:
  Volatile Data Storage Read/1 -> Data Type Conversion/1
  Data Type Conversion/1 -> Basic PWM/1, Basic PWM/2

== system webserver_demo/SQLite Demo ==
  SQLite Database Query : amg_sqlite_dataserver/SQLite Database Query  Priority=1  transfer=Non-Blocking  statement=CREATE  filenameoption=Specific  filename='database.db'  tablenameoption=Specific  tablename='sensors'  columns='pwm numeric, adc real'  condition='where rowid==1'  preview=CREATE TABLE IF NOT EXISTS %s(pwm numeric, adc real);  enablestatus=on  columncount=2  columnnamesarray="[\"pwm\",\"adc\"]"  columntypesarray="[\"uint32\",\"single\"]"  inputtypearray=[]  outputtypearray=[7]  sampletime=inf  sampletimestr=0.001  blockid=SQLiteDemoSQLiteDatabaseQuery
  SQLite Database Query1 : amg_sqlite_dataserver/SQLite Database Query  Priority=1  transfer=Non-Blocking  statement=INSERT  filenameoption=Specific  filename='database.db'  tablenameoption=Specific  tablename='sensors'  columns='pwm numeric, adc real'  condition='where rowid==1'  preview=INSERT INTO %s (pwm,adc)VALUES(%u,%f);  enablestatus=on  columncount=2  columnnamesarray="[\"pwm\",\"adc\"]"  columntypesarray="[\"uint32\",\"single\"]"  inputtypearray=[7 1]  outputtypearray=[7]  sampletime=2  sampletimestr=2  blockid=SQLiteDemoSQLiteDatabaseQuery1
  Terminator : Terminator
  Terminator1 : Terminator
  Volatile Data Storage Read : S-Function  FunctionName=waijung_vdata_read  Parameters=storagename,varname,sampletime,sampletimestr,blockid,storagetype,storagetypestr  EnableBusSupport=off  mask(waijung_vdata_read){storagename=pwm, varname=PWMDemoVolatileDataStorage_pwm, sampletime=inf, sampletimestr=2, blockid=SQLiteDemoVolatileDataStorageRead, storagetype=uint32, storagetypestr=uint32_t}
      mask prompts: storagename "Storage Name"; varname "Variable name"; sampletime "Sample time (sec)"; sampletimestr "Compiled sample time (sec) in string"; storagetype "Data type"; storagetypestr "Data type string"
      mask help: This block implements read data from a buffer.
      mask init:
      | waijung_vdata_read_callback('init');
      mask Help: web(fullfile(waijungdocroot,'waijung_vdata_read.htm'))
      mask StyleString: popup(adc|adc_f|button_on|button_off|btn2|btn3|btn1|dip|datetime|lcd_line2|lcd_line3|lcd_line4|lcd_line1|led1|pwm),edit,edit,edit,edit,edit,edit
      mask CallbackString: waijung_vdata_read_callback('storagename');|waijung_vdata_read_callback('varname');|waijung_vdata_read_callback('sampletime');|waijung_vdata_read_callback('sampletimestr');|waijung_vdata_read_callback('blockid');|waijung_vdata_read_callback('storagetype');|
      mask Display: text(0.05, 0.5, 'Buffer: pwm','ver','middle','hor','left');port_label('output',1,'D1(uint32)')
  Volatile Data Storage Read1 : S-Function  FunctionName=waijung_vdata_read  Parameters=storagename,varname,sampletime,sampletimestr,blockid,storagetype,storagetypestr  EnableBusSupport=off  mask(waijung_vdata_read){storagename=adc, varname=ADCDemoVolatileDataStorage2_adc, sampletime=inf, sampletimestr=2, blockid=SQLiteDemoVolatileDataStorageRead1, storagetype=single, storagetypestr=float}
      mask prompts: storagename "Storage Name"; varname "Variable name"; sampletime "Sample time (sec)"; sampletimestr "Compiled sample time (sec) in string"; storagetype "Data type"; storagetypestr "Data type string"
      mask help: This block implements read data from a buffer.
      mask init:
      | waijung_vdata_read_callback('init');
      mask Help: web(fullfile(waijungdocroot,'waijung_vdata_read.htm'))
      mask StyleString: popup(adc|adc_f|button_on|button_off|btn2|btn3|btn1|dip|datetime|lcd_line2|lcd_line3|lcd_line4|lcd_line1|led1|pwm),edit,edit,edit,edit,edit,edit
      mask CallbackString: waijung_vdata_read_callback('storagename');|waijung_vdata_read_callback('varname');|waijung_vdata_read_callback('sampletime');|waijung_vdata_read_callback('sampletimestr');|waijung_vdata_read_callback('blockid');|waijung_vdata_read_callback('storagetype');|
      mask Display: text(0.05, 0.5, 'Buffer: adc','ver','middle','hor','left');port_label('output',1,'D1(single)')
  wires:
  SQLite Database Query/1 -> Terminator/1
  SQLite Database Query1/1 -> Terminator1/1
  Volatile Data Storage Read1/1 -> SQLite Database Query1/2
  Volatile Data Storage Read/1 -> SQLite Database Query1/1

== system webserver_demo/SQLite Setup ==
  SQLite Database Setup : amg_sqlite_dataserver/SQLite Database Setup  Priority=1  port=UART6  timeout=5  buffersize=4096  reset=Software  resetport=A  resetpin=0  inputtypearray=[0]  outputtypearray=[0]  sampletime=inf  sampletimestr=0.001  blockid=SQLiteSetupSQLiteDatabaseSetup
  UART Setup : S-Function  Priority=1  FunctionName=stm32f4_usart  Parameters=configuration,uartmodule,transfer,baudrate,inputtype,outputtype,confstr,binheaderarray,binterminatorarray,asciiheader,asciiterminator,bindatalength,packetmode,varname,sampletime,sampletimestr,blockid  EnableBusSupport=off  mask(stm32f4_usart){configuration=Setup, uartmodule=6, baudrate=1000000, databits=8, parity=No, stopbit=1, remaptxpin=C6, remaprxpin=C7, flowcontrol=None, remapctspin=Not used, remaprtspin=Not used, advanceoptions=on, rxbuffersize=2048, txbuffersize=1024, transfer=Blocking, packetmode=Ascii, binheader='7E 7E', binterminator='03 03', porttype_double=1, porttype_single=0, porttype_int8=1, porttype_uint8=0, porttype_int16=0, porttype_uint16=0, porttype_int32=0, porttype_uint32=0, asciiformat='%d,%f', rx_asciiterminator=CRLF (0x0D 0x0A - "\r\n"), tx_asciiterminator=CR (0x0D - "\r"), storagename=<empty>, varname=, inputtype=[0], outputtype=[0], binheaderarray=[0], binterminatorarray=[0], bindatalength=0, asciiheader='', asciiterminator=[0], sampletime=-1, sampletimestr=0.001, blockid=SQLiteSetupUARTSetup, confstr=[ "dummy", "1", "C", "6", "1", "C", "7", "0", "*", "*", "0", "*", "*", "2", "5", "6", "2", "5", "1", "1024", "2048", "2", "6", "1000000", "8", "No", "1", "None", "USART6"], lastmodule=6}
      mask prompts: uartmodule "UART Module"; baudrate "Baud rate (bps)"; databits "Data bits"; stopbit "Stop bit"; remaptxpin "Tx Pin"; remaprxpin "Rx Pin"; flowcontrol "Hardware flow control"; remapctspin "HW Flow control, CTS Pin"; remaprtspin "HW Flow control, RTS Pin"; advanceoptions "Advance options"; rxbuffersize "Rx buffer size (bytes)"; txbuffersize "Tx buffer size (bytes)"; packetmode "Packet mode"; binheader "Binary header (example: '7E 7E')"; binterminator "Binary terminator (example: '03 03')"; porttype_double "Number of data port, type DOUBLE"; porttype_single "Number of data port, type SINGLE"; porttype_int8 "Number of data port, type INT8"; porttype_uint8 "Number of data port, type UINT8"; porttype_int16 "Number of data port, type INT16"; porttype_uint16 "Number of data port, type UINT16"; porttype_int32 "Number of data port, type INT32"; porttype_uint32 "Number of data port, type UINT32"; asciiformat "Ascii format"; rx_asciiterminator "End of packet"; tx_asciiterminator "End of packet"; storagename "Buffer"; varname "Var name"; inputtype "Input data type"; outputtype "Output data type"; binheaderarray "Binary header"; binterminatorarray "Binary terminator"; bindatalength "Binary data length"; asciiheader "Ascii header (printf format)"; asciiterminator "Ascii terminator"; sampletime "Sample time (sec)"; sampletimestr "Compiled sample time (sec) in string"; confstr "Configuration string"; lastmodule "Last module selected"
      mask init:
      | stm32f4_usart_callback('init');
      mask Help: web(fullfile(waijungdocroot,'stm32f4_usart_setup.htm'), '-browser')
      mask StyleString: popup(Setup|Tx|Rx),popup(1|2|3|4|5|6),edit,popup(8),popup(No|Odd|Even),popup(0.5|1|1.5|2),popup(Not used|C6|G14),popup(Not used|C7|G9),popup(None|RTS|CTS|RTS/CTS),popup(Not used|G13|G15),popup(Not used|G8|G12),checkbox,popup(16|32|64|128|256|512|1024|2048),popup(16|32|64|128|256|512|1024|2048),popup(Blocking|Non-Blocking),popup(Ascii|Binary|String Buffer),edit,edit,edit,edit,edit,edit,edit,edit,edit,edit,edit,popup(CR (0x0D - "\r")|LF (0x0A - "\n")|CRLF (0x0D 0x0A - "\r\n")),popup(CR (0x0D - "\r")|LF (0x0A - "\n")|CRLF (0x0D 0x0A - "\r\n")|None),popup(<empty>),edit,edit,edit,edit,edit,edit,edit,edit,edit,edit,edit,edit,edit
      mask CallbackString: stm32f4_usart_callback('configuration');|stm32f4_usart_callback('uartmodule');|stm32f4_usart_callback('baudrate');||||||stm32f4_usart_callback('flowcontrol');|||stm32f4_usart_callback('advanceoptions');|||stm32f4_usart_callback('transfer');|stm32f4_usart_callback('packetmode');|stm32f4_usart_callback('binheader');|stm32f4_usart_callback('binterminator');|stm32f4_usart_callback('porttype');|stm32f4_usart_callback('porttype');|stm32f4_usart_callback('porttype');|stm32f4_usart_callback('porttype');|stm32f4_usart_callback('porttype');|stm32f4_usart_callback('porttype');|stm32f4_usart_callback('porttype');|stm32f4_usart_callback('porttype');|stm32f4_usart_callback('asciiformat');|stm32f4_usart_callback('rx_asciiterminator');|stm32f4_usart_callback('tx_asciiterminator');|stm32f4_usart_callback('storagename');|stm32f4_usart_callback('varname');||||||||stm32f4_usart_callback('sampletime');|stm32f4_usart_callback('sampletimestr');|stm32f4_usart_callback('blockid');||
      mask Display: text(0.5, 0.5, 'Module: USART6_Setup\nBaud (Bps): 1000000\nDMA Buffer: 1024/2048\nTx/Rx Pin: C6/C7','ver','middle','hor','center');
